simulink library "rw_motor_torqueinput_lib"  (R2018b)
settings: Solver=VariableStepAuto  StartTime=0.0  StopTime=10.0  RelTol=1e-3
undefined symbols (not defined in the file): simParams
libraries: simulink x1
settings Model: Creator=Taylor  LastModifiedBy=Taylor

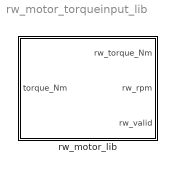
== system rw_motor_torqueinput_lib ==
  rw_motor_lib : Subsystem  mask{id_a=1}
      mask prompts: id_a "Choose the actuator ID."
      mask TypeOptions id_a: 1 | 2 | 3 | 4
      mask DialogControl DescTextVar Prompt: SOCi simplified reaction wheel model. This feeds the torque through, while integrating to get the wheel speed. If the wheel saturates, the torque is zeroed out.

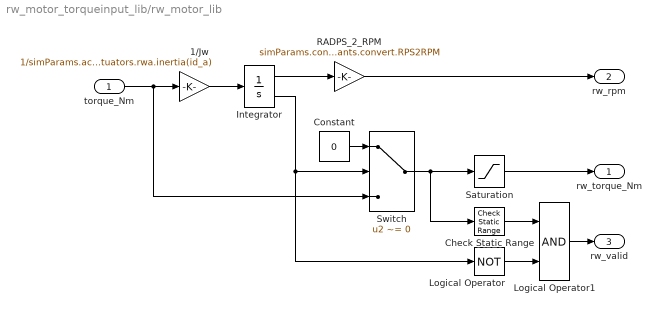
== system rw_motor_torqueinput_lib/rw_motor_lib ==
  torque_Nm : Inport
  1/Jw : Gain  Gain=1/simParams.actuators.rwa.inertia(id_a)
  Check Static Range : simulink/Model Verification/Check  Static Range  Description=-simParams.actuators.rwa.max_torque_Nm <= u <= simParams.actuators.rwa.max_torque_Nm  max=simParams.actuators.rwa.max_torque_Nm  max_included=on  min=-simParams.actuators.rwa.max_torque_Nm  min_included=on  enabled=on  stopWhenAssertionFail=off  export=on  icon=graphic
      settings: SourceProductName=Simulink  SourceProductBaseCode=SL
  Constant : Constant  Value=0
  Integrator : Integrator  InitialCondition=simParams.actuators.rwa.ic.radps(id_a)  LimitOutput=on  UpperSaturationLimit=simParams.actuators.rwa.max_RADPS  LowerSaturationLimit=-simParams.actuators.rwa.max_RADPS  ShowSaturationPort=on
  Logical Operator : Logic  Operator=NOT  AllPortsSameDT=off  OutDataTypeStr=boolean
  Logical Operator1 : Logic  AllPortsSameDT=off  OutDataTypeStr=boolean
  RADPS_2_RPM : Gain  Gain=simParams.constants.convert.RPS2RPM
  Saturation : Saturate  UpperLimit=simParams.actuators.rwa.max_torque_Nm  LowerLimit=-simParams.actuators.rwa.max_torque_Nm  ZeroCross=off
  Switch : Switch  Criteria=u2 ~= 0
  rw_torque_Nm : Outport
  rw_rpm : Outport  Port=2
  rw_valid : Outport  Port=3
  wires:
  1/Jw/1 -> Integrator/1
  torque_Nm/1 -> Switch/3, 1/Jw/1
  Integrator/1 -> RADPS_2_RPM/1
  RADPS_2_RPM/1 -> rw_rpm/1
  Integrator/2 -> Logical Operator/1, Switch/2
  Constant/1 -> Switch/1
  Switch/1 -> Check Static Range/1, Saturation/1
  Saturation/1 -> rw_torque_Nm/1
  Check Static Range/1 -> Logical Operator1/1
  Logical Operator/1 -> Logical Operator1/2
  Logical Operator1/1 -> rw_valid/1
